simulink model "ESP32_UDP_UART_Bridge"  (R2024b)
settings: Solver=ode4  StartTime=0.0  StopTime=Inf  FixedStep=0.005  RelTol=1e-3  EnableMultiTasking=on
values from neighbouring files (symbols this model uses):
  UDP_DIAG_SOURCE_ID = uint8(1)    [ESP32_UDP_UART_Setup.m]
libraries: arduinowifilib x1, arduinolib x1
(part 3 of 3)

== matlab function ESP32_UDP_UART_Bridge/MATLAB Function ==
  data: now_ms input; portA_status_u8 input; portA_time_u32 input; portA_pose_f32 input; portB_status_u8 input; portB_time_u32 input; portB_pose_f32 input; src_status_u8 output; scenario input; src_time_u32 output; src_pose_f32 output
function [src_status_u8, src_time_u32, src_pose_f32] = Vision_Source_Memory(now_ms, ...
    portA_status_u8, portA_time_u32, portA_pose_f32, ...
    portB_status_u8, portB_time_u32, portB_pose_f32, ...
    scenario)
%#codegen
% =========================================================
% Vision_Source_Memory
% =========================================================
% Zadanie:
%   Buforuje ostatni stan każdego źródła Vision source_id=1..4.
%   Blok może pracować w dwóch trybach:
%
%   scenario = 0:
%       tryb normalny, dane idą z dekoderów ATB1/UDP.
%
%   scenario = 1..3:
%       tryb testowy, blok ignoruje wejścia z dekoderów i sam generuje
%       syntetyczne ramki testowe do sprawdzenia logiki wielu telefonów.
%
% Dlaczego ten blok istnieje:
%   Pozwala sprawdzić logikę Source Memory → Predictor → Fusion → Safety
%   bez prawdziwego telefonu, UDP i CRC. Dzięki temu można przetestować
%   problem: jeden telefon trzyma deadman, drugi jest obserwatorem albo
%   widzi tylko bazę i ma valid=0/deadman=0.
%
% Wejścia normalne:
%   now_ms              : lokalny czas ESP32 w ms, uint32
%   portA_status_u8     : status z dekodera PortA/UDP 5005
%   portA_time_u32      : seq i unity_t_ms z dekodera PortA
%   portA_pose_f32      : pozycja/yaw z dekodera PortA
%   portB_status_u8     : status z dekodera PortB/UDP 5006
%   portB_time_u32      : seq i unity_t_ms z dekodera PortB
%   portB_pose_f32      : pozycja/yaw z dekodera PortB
%   scenario            : 0=real UDP, 1..3=testy
%
% Wyjścia:
%   src_status_u8, 8x4:
%     kolumny = source_id 1..4
%     1 = seen
%     2 = has_pose
%     3 = valid
%     4 = deadman
%     5 = move_en
%     6 = speed_pct
%     7 = fps_hz
%     8 = last_rx_port_id, 1=PortA/5005, 2=PortB/5006
%
%   src_time_u32, 5x4:
%     1 = seq
%     2 = unity_t_ms
%     3 = last_frame_rx_ms
%     4 = last_pose_rx_ms
%     5 = prev_pose_rx_ms
%
%   src_pose_f32, 10x4:
%     1  = x_last
%     2  = y_last
%     3  = z_last
%     4  = yaw_deg_last
%     5  = yaw_unwrapped_last
%     6  = yaw_rate_dps
%     7  = x_prev
%     8  = y_prev
%     9  = z_prev
%     10 = yaw_unwrapped_prev
%
% Scenariusze testowe:
%   scenario=1:
%     source 1: valid=1, deadman=1, move_en=1, daje pozycję
%     source 2: valid=0, deadman=0, move_en=0, obserwator/brak auta
%     Oczekiwane:
%       operator_enable_sources_mask = 1
%       candidate_sources_mask = 1
%       fused_available = 1
%       hard_stop = 0
%
%   scenario=2:
%     source 1: valid=0, deadman=1, move_en=1, tylko zgoda na jazdę
%     source 2: valid=1, deadman=0, move_en=0, tylko pozycja
%     Oczekiwane:
%       operator_enable_sources_mask = 1
%       candidate_sources_mask = 2
%       fused_source_id = 2
%       speed_pct z source 1
%       hard_stop = 0
%
%   scenario=3:
%     brak źródła z deadman=1 i move_en=1
%     Oczekiwane:
%       operator_enable_sources_mask = 0
%       operator_stop_request = 1
%       hard_stop = 1
% =========================================================

persistent status_buf time_buf pose_buf last_scenario

sc = uint8(scenario);

if isempty(status_buf)
    status_buf = zeros(8, 4, 'uint8');
    time_buf   = zeros(5, 4, 'uint32');
    pose_buf   = zeros(10, 4, 'single');
    last_scenario = sc;
end

% Reset bufora przy starcie symulacji albo zmianie scenariusza.
% Dzięki temu stare dane z poprzedniego scenariusza nie mieszają testów.
if now_ms == uint32(0) || sc ~= last_scenario
    status_buf = zeros(8, 4, 'uint8');
    time_buf   = zeros(5, 4, 'uint32');
    pose_buf   = zeros(10, 4, 'single');
    last_scenario = sc;
end

% Lokalne ramki, które potem aktualizują wspólny bufor.
A_status = portA_status_u8;
A_time   = portA_time_u32;
A_pose   = portA_pose_f32;

B_status = portB_status_u8;
B_time   = portB_time_u32;
B_pose   = portB_pose_f32;

% scenario=0: realne dane z dekoderów.
% scenario>0: nadpisujemy lokalne A/B danymi testowymi.
if sc ~= uint8(0)
    [A_status, A_time, A_pose, B_status, B_time, B_pose] = build_test_frames(now_ms, sc);
end

% PortA = 1, zwykle UDP 5005
[status_buf, time_buf, pose_buf] = update_source(now_ms, uint8(1), A_status, A_time, A_pose, status_buf, time_buf, pose_buf);

% PortB = 2, zwykle UDP 5006
[status_buf, time_buf, pose_buf] = update_source(now_ms, uint8(2), B_status, B_time, B_pose, status_buf, time_buf, pose_buf);

src_status_u8 = status_buf;
src_time_u32  = time_buf;
src_pose_f32  = pose_buf;
end

function [A_status, A_time, A_pose, B_status, B_time, B_pose] = build_test_frames(now_ms, sc)
%#codegen

A_status = zeros(8, 1, 'uint8');
A_time   = zeros(2, 1, 'uint32');
A_pose   = zeros(6, 1, 'single');

B_status = zeros(8, 1, 'uint8');
B_time   = zeros(2, 1, 'uint32');
B_pose   = zeros(6, 1, 'single');

t_s = single(double(now_ms) / 1000.0);
seq = uint32(double(now_ms) / 50.0);

if sc == uint8(1)
    % =====================================================
    % Scenario 1
    % Source 1: pozycja + deadman
    % Source 2: obserwator, valid=0, deadman=0
    % =====================================================

    A_status(1) = uint8(1);  % frame_ok
    A_status(2) = uint8(1);  % source_id
    A_status(3) = uint8(1);  % valid
    A_status(4) = uint8(1);  % deadman
    A_status(5) = uint8(1);  % move_en
    A_status(6) = uint8(50); % speed_pct
    A_status(7) = uint8(20); % fps_hz
    A_status(8) = uint8(0);  % reserved

    A_time(1) = seq;
    A_time(2) = now_ms;

    A_pose(1) = single(0.40) + single(0.10) * t_s;
    A_pose(2) = single(0.20);
    A_pose(3) = single(0.00);
    A_pose(4) = single(90.0);
    A_pose(5) = single(90.0);
    A_pose(6) = single(0.0);

    B_status(1) = uint8(1);  % frame_ok
    B_status(2) = uint8(2);  % source_id
    B_status(3) = uint8(0);  % valid=0
    B_status(4) = uint8(0);  % deadman=0
    B_status(5) = uint8(0);  % move_en=0
    B_status(6) = uint8(0);
    B_status(7) = uint8(20);
    B_status(8) = uint8(0);

    B_time(1) = seq;
    B_time(2) = now_ms;

elseif sc == uint8(2)
    % =====================================================
    % Scenario 2
    % Source 1: tylko deadman/move_en, bez pozycji
    % Source 2: tylko pozycja, bez deadmana
    % =====================================================

    A_status(1) = uint8(1);  % frame_ok
    A_status(2) = uint8(1);  % source_id
    A_status(3) = uint8(0);  % valid=0, brak pozycji
    A_status(4) = uint8(1);  % deadman=1
    A_status(5) = uint8(1);  % move_en=1
    A_status(6) = uint8(40); % speed_pct
    A_status(7) = uint8(20);
    A_status(8) = uint8(0);

    A_time(1) = seq;
    A_time(2) = now_ms;

    B_status(1) = uint8(1);  % frame_ok
    B_status(2) = uint8(2);  % source_id
    B_status(3) = uint8(1);  % valid=1, pozycja
    B_status(4) = uint8(0);  % deadman=0
    B_status(5) = uint8(0);  % move_en=0
    B_status(6) = uint8(0);
    B_status(7) = uint8(20);
    B_status(8) = uint8(0);

    B_time(1) = seq;
    B_time(2) = now_ms;

    B_pose(1) = single(0.50) + single(0.10) * t_s;
    B_pose(2) = single(0.25);
    B_pose(3) = single(0.00);
    B_pose(4) = single(92.0);
    B_pose(5) = single(92.0);
    B_pose(6) = single(0.0);

else
    % =====================================================
    % Scenario 3
    % Brak operator_enable, czyli deadman/move_en puszczone
    % =====================================================

    A_status(1) = uint8(1);  % frame_ok
    A_status(2) = uint8(1);  % source_id
    A_status(3) = uint8(1);  % valid=1
    A_status(4) = uint8(0);  % deadman=0
    A_status(5) = uint8(0);  % move_en=0
    A_status(6) = uint8(0);
    A_status(7) = uint8(20);
    A_status(8) = uint8(0);

    A_time(1) = seq;
    A_time(2) = now_ms;

    A_pose(1) = single(0.40);
    A_pose(2) = single(0.20);
    A_pose(3) = single(0.00);
    A_pose(4) = single(90.0);
    A_pose(5) = single(90.0);
    A_pose(6) = single(0.0);
end
end

function [status_buf, time_buf, pose_buf] = update_source(now_ms, rx_port_id, rx_status_u8, rx_time_u32, rx_pose_f32, status_buf, time_buf, pose_buf)
%#codegen

frame_ok = rx_status_u8(1);

if frame_ok == 0
    return;
end

source_id = rx_status_u8(2);

if source_id < uint8(1) || source_id > uint8(4)
    return;
end

idx = double(source_id);
valid = rx_status_u8(3);

% seen
status_buf(1, idx) = uint8(1);

% last_frame_rx_ms
time_buf(3, idx) = now_ms;

% status
status_buf(3, idx) = rx_status_u8(3); % valid
status_buf(4, idx) = rx_status_u8(4); % deadman
status_buf(5, idx) = rx_status_u8(5); % move_en
status_buf(6, idx) = rx_status_u8(6); % speed_pct
status_buf(7, idx) = rx_status_u8(7); % fps_hz

% Diagnostyka portu fizycznego:
% 1 = PortA / zwykle UDP 5005
% 2 = PortB / zwykle UDP 5006
status_buf(8, idx) = rx_port_id;

% time
time_buf(1, idx) = rx_time_u32(1); % seq
time_buf(2, idx) = rx_time_u32(2); % unity_t_ms

% Pozycję aktualizujemy tylko przy valid=1.
% valid=0 aktualizuje status/deadman/move_en, ale nie nadpisuje pozycji.
if valid ~= 0

    has_pose = status_buf(2, idx);

    if has_pose ~= 0
        time_buf(5, idx) = time_buf(4, idx); % prev_pose_rx_ms

        pose_buf(7, idx)  = pose_buf(1, idx); % x_prev
        pose_buf(8, idx)  = pose_buf(2, idx); % y_prev
        pose_buf(9, idx)  = pose_buf(3, idx); % z_prev
        pose_buf(10, idx) = pose_buf(5, idx); % yaw_unwrapped_prev
    else
        time_buf(5, idx) = now_ms;

        pose_buf(7, idx)  = rx_pose_f32(1);
        pose_buf(8, idx)  = rx_pose_f32(2);
        pose_buf(9, idx)  = rx_pose_f32(3);
        pose_buf(10, idx) = rx_pose_f32(5);
    end

    status_buf(2, idx) = uint8(1); % has_pose

    time_buf(4, idx) = now_ms; % last_pose_rx_ms

    pose_buf(1, idx) = rx_pose_f32(1); % x_last
    pose_buf(2, idx) = rx_pose_f32(2); % y_last
    pose_buf(3, idx) = rx_pose_f32(3); % z_last
    pose_buf(4, idx) = rx_pose_f32(4); % yaw_deg_last
    pose_buf(5, idx) = rx_pose_f32(5); % yaw_unwrapped_last
    pose_buf(6, idx) = rx_pose_f32(6); % yaw_rate_dps
end
end
